simulink model "Copy_of_Pacemaker_images"  (R2022a)
settings: Solver=FixedStepAuto  StartTime=0.0  StopTime=40  FixedStep=1e-3  RelTol=1e-3  EnableMultiTasking=on
undefined symbols (not defined in the file or in its folder): ARP, ATR_Amplitude, ATR_CMP_DETECT, ATR_Pulse_Width, ATR_Sensitivity, D10, D11, D12, D13, D2, D3, D4, D5, D6, D7, D8, D9, Hecate_delayEnd, Hecate_delayOff, Hecate_DELAYOFF, Hecate_delayOn, Hecate_DELAYON, Hecate_HEARTFAIL, Hecate_MODE, LRL, Mode, PTA0, PTA1, PTA2, PTB23, PTB9, PTC2, PTC3, PTC4, PTD0, PTD1, PTD2, PTD3, VENT_Amplitude, VENT_CMP_DETECT, VENT_Pulse_Width, VENT_Sensitivity, VRP
libraries: frdmk64flib x15
settings Model: ExtModeTrigDuration=5  Creator=akshayjacob  LastModifiedBy=fedformi_new
settings DataIOCC: SaveFormat=Array  ReturnWorkspaceOutputs=off
settings OptimizationCC: DefaultParameterBehavior=Inlined  EnhancedBackFolding=on  PassReuseOutputArgsAs=Individual arguments  ZeroExternalMemoryAtStartup=off  ZeroInternalMemoryAtStartup=off  MaxStackSize=64  OptimizeBlockOrder=speed  DifferentSizesBufferReuse=on  OptimizationCustomize=off  EfficientTunableParamExpr=on
settings DebuggingCC: ParameterTunabilityLossMsg=error  UnconnectedInputMsg=warning  UnconnectedOutputMsg=warning  UnconnectedLineMsg=warning
settings HardwareCC: ProdBitPerPointer=32  ProdBitPerSizeT=32  ProdBitPerPtrDiffT=32  ProdLargestAtomicInteger=Long  ProdLargestAtomicFloat=Double  ProdWordSize=32  ProdHWDeviceType=ARM Compatible->ARM Cortex
settings SFSimCC: MATLABDynamicMemAlloc=off
settings RTWCC: SystemTargetFile=ert.tlc  TemplateMakefile=ert_default_tmf  Toolchain=GNU Tools for ARM Embedded Processors  DLArmComputeVersion=19.05
settings CodeAppCC: ForceParamTrailComments=on  IgnoreCustomStorageClasses=off  OperatorAnnotations=on  SimulinkDataObjDesc=on  SFDataObjDesc=on  InsertBlockDesc=on
settings ERTTargetCC: ERTCustomFileTemplate=example_file_process.tlc

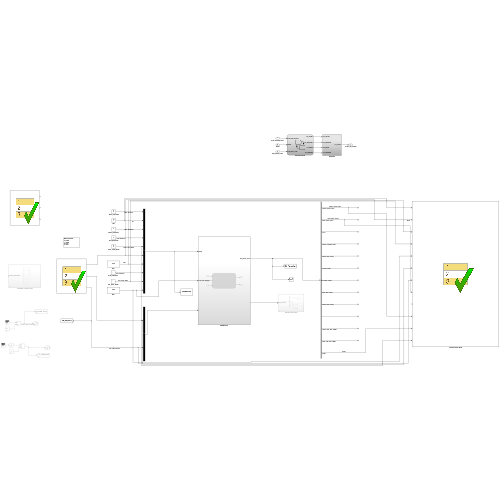
[thumbnail: Simulink's stored preview of the top-level diagram]
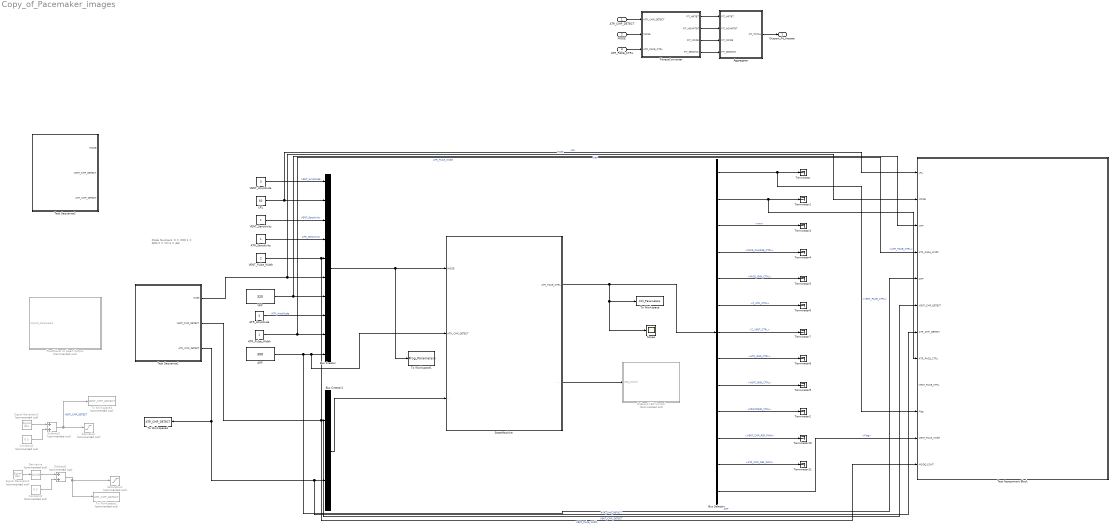
== system Copy_of_Pacemaker_images ==
  note: Mode Numbers:
      |
      | 0 = VOO
      | 1 = AOO
      | 2 = VVI
      | 3 = AAI
  ATR_CMP_DETECT : Inport
  MODE : Inport  Port=2
  ATR_PACE_CTRL : Inport  Port=3
  ARP : Constant  Value=300
  ATR_Amplitude : Constant  Value=3
  ATR_Pulse_Width : Constant
  ATR_Sensitivity : Constant
  Aggregator : Subsystem
  Bus Creator : BusCreator  Inputs=VENT_Amplitude,LRL,VENT_Sensitivity,ATR_Sensitivity,VENT_Pulse_Width,Mode,VRP,ATR_Amplitude,ATR_Pulse_Width,ARP
  Bus Creator1 : BusCreator  Inputs=VENT_CMP_DETECT,ATR_CMP_DETECT
  Bus Selector : BusSelector  OutputSignals=VENT_PACE_CTRL,ATR_PACE_CTRL,nnn,PACE_CHARGE_CTRL,PACE_GND_CTRL,Z_ATR_CTRL,Z_VENT_CTRL,ATR_GND_CTRL,VENT_GND_CTRL,FRONTEND_CTRL,VENT_CMP_REF_PWM,ATR_CMP_REF_PWM,Flag
  Constant1 : Constant  Commented=on  Value=0.5
  Constant2 : Constant  Commented=on  Value=0.5
  Derivative : Derivative  Commented=on
  FitnessConverter : Stateflow chart  TreatAsAtomicUnit=on
  LRL : Constant  Value=60
  OnBoard LED Control : Subsystem  Commented=on
  PaceMaker to Heart Output : Subsystem  Commented=on
  Saturation : Saturate  Commented=on  UpperLimit=1  LowerLimit=0
  Saturation1 : Saturate  Commented=on  UpperLimit=1  LowerLimit=0
  Scope : Scope
  Signal Generator1 : SignalGenerator  Commented=on  Amplitude=1.5  Frequency=1/5
  Signal Generator2 : SignalGenerator  Commented=on  Amplitude=1.5  Frequency=1/5
  StateMachine : Subsystem
  Subtract1 : Sum  Commented=on
  Subtract2 : Sum  Commented=on
  Terminator{,1..11} (12 alike) : Terminator
  Test Assessment Block : Test Sequence  Tag=__SLT_ASMT__  TreatAsAtomicUnit=on
  Test Sequence1 : Test Sequence  TreatAsAtomicUnit=on
  Test Sequence2 : Test Sequence  TreatAsAtomicUnit=on
  To Workspace : ToWorkspace  VariableName=Ctrl_Parameters  SaveFormat=Timeseries  SampleTime=-1
  To Workspace1 : ToWorkspace  VariableName=Prog_Parameters  SaveFormat=Timeseries  SampleTime=-1
  To Workspace2 : ToWorkspace  Commented=on  VariableName=ATR_CMP_DETECT  SaveFormat=Timeseries  SampleTime=-1
  To Workspace3 : ToWorkspace  Commented=on  VariableName=VENT_CMP_DETECT  SaveFormat=Timeseries  SampleTime=-1
  To Workspace4 : ToWorkspace  VariableName=ATR_CMP_DETECT  SaveFormat=Timeseries  SampleTime=-1
  VENT_Amplitude : Constant  Value=3
  VENT_Pulse_Width : Constant  Value=2
  VENT_Sensitivity : Constant
  VRP : Constant  Value=320
  Outport_Fit_Hecate : Outport
  wires:
  Bus Creator/1 -> To Workspace1/1, StateMachine/1(MODE)
  StateMachine/2(.  .  .) -> OnBoard LED Control/1(LED_Control)
  Bus Creator1/1 -> StateMachine/3(. . .)
  VRP/1 -> Test Assessment Block/3(VRP), Bus Creator/7  "VRP"
  ATR_Sensitivity/1 -> Bus Creator/4  "ATR_Sensitivity"
  ATR_Pulse_Width/1 -> Test Assessment Block/4(ATR_Pulse_Width), Bus Creator/9  "ATR_Pulse_Width"
  LRL/1 -> Test Assessment Block/1(LRL), Bus Creator/2  "LRL"
  ATR_Amplitude/1 -> Bus Creator/8  "ATR_Amplitude"
  ARP/1 -> Test Assessment Block/5(ARP), StateMachine/2(ATR_CMP_DETECT), Bus Creator/10  "ARP"
  VENT_Sensitivity/1 -> Bus Creator/3  "VENT_Sensitivity"
  VENT_Amplitude/1 -> Bus Creator/1  "VENT_Amplitude"
  VENT_Pulse_Width/1 -> Test Assessment Block/12(MODE_CONT), Bus Creator/5  "VENT_Pulse_Width"
  Test Sequence1/1(Mode) -> Test Assessment Block/2(MODE), Bus Creator/6  "Mode"
  Subtract1/1 -> Saturation1/1, To Workspace2/1
  Signal Generator2/1 -> Subtract2/1
  Test Sequence1/2(VENT_CMP_DETECT) -> Test Assessment Block/6(VENT_CMP_DETECT), Bus Creator1/1  "VENT_CMP_DETECT"
  Constant1/1 -> Subtract1/2
  Constant2/1 -> Subtract2/2
  Test Sequence1/3(ATR_CMP_DETECT) -> To Workspace4/1, Bus Creator1/2, Test Assessment Block/7(ATR_CMP_DETECT)  "ATR_CMP_DETECT"
  Subtract2/1 -> Saturation/1, To Workspace3/1  "VENT_CMP_DETECT"
  Derivative/1 -> Subtract1/1
  Signal Generator1/1 -> Derivative/1
  Bus Selector/12 -> Terminator11/1  "<ATR_CMP_REF_PWM>"
  Bus Selector/3 -> Terminator3/1  "<nnn>"
  Bus Selector/7 -> Terminator7/1  "<Z_VENT_CTRL>"
  Bus Selector/10 -> Terminator2/1  "<FRONTEND_CTRL>"
  Bus Selector/8 -> Terminator8/1  "<ATR_GND_CTRL>"
  StateMachine/1(ATR_PACE_CTRL) -> Bus Selector/1, Scope/1, To Workspace/1
  Bus Selector/1 -> Test Assessment Block/10(Flag), Terminator/1  "<VENT_PACE_CTRL>"
  Bus Selector/5 -> Terminator5/1  "<PACE_GND_CTRL>"
  Bus Selector/9 -> Terminator9/1  "<VENT_GND_CTRL>"
  Bus Selector/2 -> Test Assessment Block/8(ATR_PACE_CTRL), Terminator1/1  "<ATR_PACE_CTRL>"
  Bus Selector/11 -> Terminator10/1  "<VENT_CMP_REF_PWM>"
  Bus Selector/6 -> Terminator6/1  "<Z_ATR_CTRL>"
  Bus Selector/4 -> Terminator4/1  "<PACE_CHARGE_CTRL>"
  Bus Selector/13 -> Test Assessment Block/11(VENT_Pulse_Width)  "<Flag>"
  FitnessConverter/2(FIT_NOHRTBT) -> Aggregator/2(FIT_NOHRTBT)
  FitnessConverter/3(FIT_MODE) -> Aggregator/3(FIT_MODE)
  Aggregator/1(FIT_TOTAL) -> Outport_Fit_Hecate/1
  FitnessConverter/1(FIT_HRTBT) -> Aggregator/1(FIT_HRTBT)
  FitnessConverter/4(FIT_SENSING) -> Aggregator/4(FIT_SENSING)
  ATR_CMP_DETECT/1 -> FitnessConverter/1(ATR_CMP_DETECT)
  MODE/1 -> FitnessConverter/2(MODE)
  ATR_PACE_CTRL/1 -> FitnessConverter/3(ATR_PACE_CTRL)

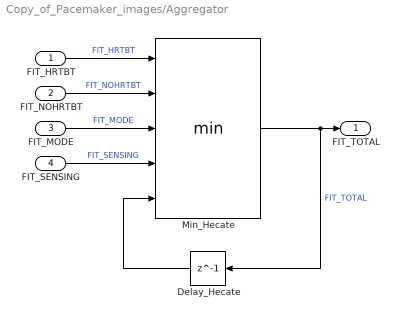
== system Copy_of_Pacemaker_images/Aggregator ==
  FIT_HRTBT : Inport
  FIT_NOHRTBT : Inport  Port=2
  FIT_MODE : Inport  Port=3
  FIT_SENSING : Inport  Port=4
  Delay_Hecate : Delay  DelayLength=1  InitialCondition=Inf
  Min_Hecate : MinMax  Inputs=5
  FIT_TOTAL : Outport
  wires:
  FIT_NOHRTBT/1 -> Min_Hecate/2  "FIT_NOHRTBT"
  FIT_MODE/1 -> Min_Hecate/3  "FIT_MODE"
  Delay_Hecate/1 -> Min_Hecate/5
  FIT_HRTBT/1 -> Min_Hecate/1  "FIT_HRTBT"
  Min_Hecate/1 -> FIT_TOTAL/1, Delay_Hecate/1  "FIT_TOTAL"
  FIT_SENSING/1 -> Min_Hecate/4  "FIT_SENSING"

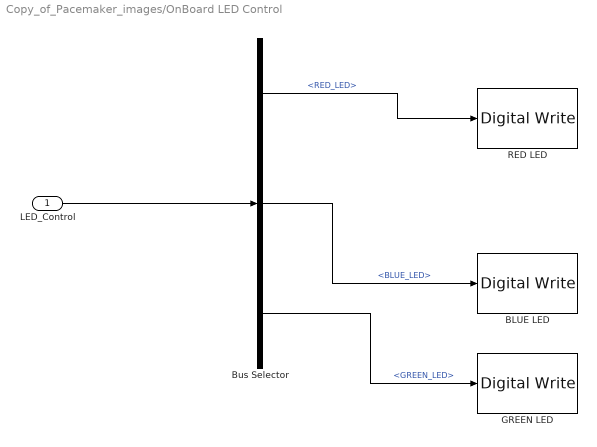
== system Copy_of_Pacemaker_images/OnBoard LED Control ==
  LED_Control : Inport
  BLUE LED : frdmk64flib/Digital Write  Whichpin=BLUE_LED
  Bus Selector : BusSelector  OutputSignals=RED_LED,BLUE_LED,GREEN_LED
  GREEN LED : frdmk64flib/Digital Write  Whichpin=GREEN_LED
  RED LED : frdmk64flib/Digital Write  Whichpin=RED_LED
  wires:
  LED_Control/1 -> Bus Selector/1
  Bus Selector/1 -> RED LED/1  "<RED_LED>"
  Bus Selector/2 -> BLUE LED/1  "<BLUE_LED>"
  Bus Selector/3 -> GREEN LED/1  "<GREEN_LED>"

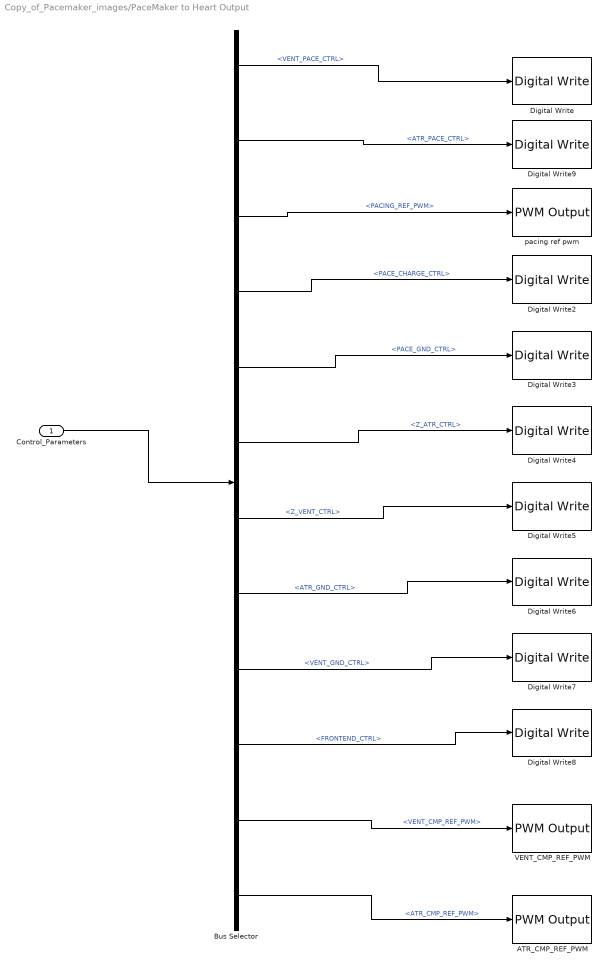
== system Copy_of_Pacemaker_images/PaceMaker to Heart Output ==
  Control_Parameters : Inport
  ATR_CMP_REF_PWM : frdmk64flib/PWM Output  Whichpin=PTC2 (D6)  InitialFrequency=2000  InitialDutyCycle=0
  Bus Selector : BusSelector  OutputSignals=VENT_PACE_CTRL,ATR_PACE_CTRL,PACING_REF_PWM,PACE_CHARGE_CTRL,PACE_GND_CTRL,Z_ATR_CTRL,Z_VENT_CTRL,ATR_GND_CTRL,VENT_GND_CTRL,FRONTEND_CTRL,VENT_CMP_REF_PWM,ATR_CMP_REF_PWM
  Digital Write : frdmk64flib/Digital Write  Whichpin=PTC4 (D9)
  Digital Write2 : frdmk64flib/Digital Write  Whichpin=PTB9 (D2)
  Digital Write3 : frdmk64flib/Digital Write  Whichpin=PTD0 (D10)
  Digital Write4 : frdmk64flib/Digital Write  Whichpin=PTB23 (D4)
  Digital Write5 : frdmk64flib/Digital Write  Whichpin=PTC3 (D7)
  Digital Write6 : frdmk64flib/Digital Write  Whichpin=PTD2 (D11)
  Digital Write7 : frdmk64flib/Digital Write  Whichpin=PTD3 (D12)
  Digital Write8 : frdmk64flib/Digital Write  Whichpin=PTD1 (D13)
  Digital Write9 : frdmk64flib/Digital Write  Whichpin=PTA0 (D8)
  VENT_CMP_REF_PWM : frdmk64flib/PWM Output  Whichpin=PTA1 (D3)  InitialFrequency=2000  InitialDutyCycle=0
  pacing ref pwm : frdmk64flib/PWM Output  Whichpin=PTA2 (D5)  InitialFrequency=2000  InitialDutyCycle=0
  wires:
  Control_Parameters/1 -> Bus Selector/1
  Bus Selector/1 -> Digital Write/1  "<VENT_PACE_CTRL>"
  Bus Selector/3 -> pacing ref pwm/1  "<PACING_REF_PWM>"
  Bus Selector/4 -> Digital Write2/1  "<PACE_CHARGE_CTRL>"
  Bus Selector/5 -> Digital Write3/1  "<PACE_GND_CTRL>"
  Bus Selector/6 -> Digital Write4/1  "<Z_ATR_CTRL>"
  Bus Selector/7 -> Digital Write5/1  "<Z_VENT_CTRL>"
  Bus Selector/8 -> Digital Write6/1  "<ATR_GND_CTRL>"
  Bus Selector/9 -> Digital Write7/1  "<VENT_GND_CTRL>"
  Bus Selector/10 -> Digital Write8/1  "<FRONTEND_CTRL>"
  Bus Selector/2 -> Digital Write9/1  "<ATR_PACE_CTRL>"
  Bus Selector/11 -> VENT_CMP_REF_PWM/1  "<VENT_CMP_REF_PWM>"
  Bus Selector/12 -> ATR_CMP_REF_PWM/1  "<ATR_CMP_REF_PWM>"

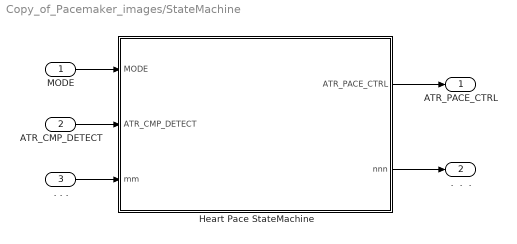
== system Copy_of_Pacemaker_images/StateMachine ==
  MODE : Inport
  ATR_CMP_DETECT : Inport  Port=2
  . . . : Inport  Port=3
  Heart Pace StateMachine : Stateflow chart  TreatAsAtomicUnit=on
  ATR_PACE_CTRL : Outport
  .  .  . : Outport  Port=2
  wires:
  MODE/1 -> Heart Pace StateMachine/1(MODE)
  ATR_CMP_DETECT/1 -> Heart Pace StateMachine/2(ATR_CMP_DETECT)
  . . ./1 -> Heart Pace StateMachine/3(mm)
  Heart Pace StateMachine/1(ATR_PACE_CTRL) -> ATR_PACE_CTRL/1
  Heart Pace StateMachine/2(nnn) -> .  .  ./1

== stateflow chart Copy_of_Pacemaker_images/FitnessConverter ==
  state MODE_SELECTION
    FIT_HRTBT = Inf;
    FIT_NOHRTBT = Inf;
    FIT_MODE = Inf;
    FIT_SENSING = Inf;
    state MODE_3
      FIT_HRTBT = Inf;
      FIT_NOHRTBT = Inf;
      FIT_MODE = Inf;
      FIT_SENSING = Inf;
      state NO_HEARTBEAT
        FIT_HRTBT = Inf;
        FIT_NOHRTBT = 0-(et);
        FIT_MODE = Inf;
        FIT_SENSING = Inf;
      state HEARTBEAT
        FIT_HRTBT = 1;
        FIT_NOHRTBT = Inf;
        FIT_MODE = Inf;
        FIT_SENSING = Inf;
      state SENSING
        FIT_HRTBT = Inf;
        FIT_NOHRTBT = Inf;
        FIT_MODE = Inf;
        FIT_SENSING = 60/LRL-et;
      (default) -> SENSING
      NO_HEARTBEAT -> SENSING : [ATR_CMP_DETECT == true || ...
          |  ATR_PACE_CTRL == true]
      SENSING -> NO_HEARTBEAT [order 2] : [et > 60/LRL]
      SENSING -> HEARTBEAT [order 1] : [ATR_CMP_DETECT == true || ...
          |  ATR_PACE_CTRL == true]
      HEARTBEAT -> SENSING : [true]
    state ELSE
      FIT_HRTBT = Inf;
      FIT_NOHRTBT = Inf;
      FIT_MODE = 3.5-(MODE_CONT);
      FIT_SENSING = Inf;
    (default) -> (junction 4)
    (junction 4) -> ELSE [order 2]
    (junction 4) -> MODE_3 [order 1] : [(MODE == 3)]
    ELSE -> (junction 4) : [((MODE == 3))]
    MODE_3 -> (junction 4) : [~((MODE == 3))]
  (default) -> MODE_SELECTION
  data: ATR_CMP_DETECT input; MODE input; ATR_PACE_CTRL input; FIT_HRTBT output; FIT_NOHRTBT output; FIT_MODE output; MODE_CONT local; LRL local; FIT_SENSING output

== stateflow chart Copy_of_Pacemaker_images/Test Assessment Block ==
  state Complete
    state Run
      state AAI
        state AAI_Refractory
          verify(ATR_PACE_CTRL==0)
          settings: description=|
              | after(ARP-(ATR_Pulse_Width ...
              | *Flag),msec)
        state AAI_Sensing
          verify(ATR_PACE_CTRL==0)
          settings: description=after(60000/LRL-ARP, msec)
        state AAI_Pacing
          verify(ATR_PACE_CTRL==1);
          settings: description=after(ATR_Pulse_Width,msec)
        AAI_Pacing -> (junction 603) : [
            | et > (ATR_Pulse_Width)/1000
            | ]
        (default) -> AAI_Refractory
        (junction 601) -> AAI_Refractory
        AAI_Refractory -> AAI_Sensing : [
            | et > (ARP-(ATR_Pulse_Width ...
            | *Flag))/1000
            | ]
        AAI_Sensing -> AAI_Refractory [order 1] : [
            | [(ATR_CMP_DETECT == 1)]
            | ]
        AAI_Sensing -> AAI_Pacing [order 2] : [
            | et > (60000/LRL-ARP)/1000
            | ]
        (junction 603) -> (junction 601)
      state VVI
        state VVI_REFRACTORY
          verify(VENT_PACE_CTRL==0);
          settings: description=after(VRP - (VENT_Pulse_Width * Flag-1),msec)
        state VVI_SENSE
          verify(VENT_PACE_CTRL==0);
          settings: description=after(60000/LRL - VRP, msec)
        state VVI_PACING
          verify(VENT_PACE_CTRL==1);
          settings: description=after(VENT_Pulse_Width,msec)
        VVI_PACING -> (junction 611) : [
            | et > (VENT_Pulse_Width)/1000
            | ]
        (default) -> VVI_REFRACTORY
        (junction 609) -> VVI_REFRACTORY
        VVI_REFRACTORY -> VVI_SENSE : [
            | et > (VRP - (VENT_Pulse_Width * Flag-1))/1000
            | ]
        VVI_SENSE -> VVI_REFRACTORY [order 2] : [
            | VENT_CMP_DETECT == 1
            | ]
        VVI_SENSE -> VVI_PACING [order 1] : [
            | et > (60000/LRL - VRP)/1000
            | ]
        (junction 611) -> (junction 609)
      state default
      Run -> (junction 557)
      (default) -> (junction 557)
      (junction 557) -> (junction 558) [order 1] : [Mode == 3
          | ]
      (junction 558) -> AAI [order 1] : [~in(Complete.Run.AAI)]
      (junction 557) -> (junction 574) [order 2]
      (junction 558) -> (junction 561) [order 2]
      (junction 574) -> (junction 575) [order 1] : [Mode ==2
          | ]
      (junction 575) -> VVI [order 1] : [~in(Complete.Run.VVI)]
      (junction 575) -> (junction 578) [order 2]
      (junction 590) -> (junction 591)
      (junction 591) -> default [order 1] : [~in(Complete.Run.default)]
      (junction 591) -> (junction 594) [order 2]
      (junction 574) -> (junction 590) [order 2]
    (default) -> Run
  state Partial
    state Mode_selection
      state Mode_3
        state Sensing
          verify(et <= 60/LRL)
        state Heartbeat
          verify(true)
        state No_heartbeat
          verify(false)
        (junction 677) -> (junction 660)
        (default) -> Sensing
        (junction 660) -> Sensing
        Sensing -> (junction 672) [order 2] : [
            | et >= 60/LRL
            | ]
        (junction 672) -> (junction 652)
        Sensing -> Heartbeat [order 1] : [
            | ATR_CMP_DETECT == true || ...
            |  ATR_PACE_CTRL == true
            | ]
        Heartbeat -> Sensing : [
            | true
            | ]
        (junction 652) -> No_heartbeat
        No_heartbeat -> (junction 677) : [
            | ATR_CMP_DETECT == true || ...
            |  ATR_PACE_CTRL == true
            | ]
      state Else
        verify(MODE_CONT <= 3.5)
      (default) -> (junction 627)
      Mode_selection -> (junction 627)
      (junction 627) -> (junction 628) [order 1] : [(MODE == 3)
          | ]
      (junction 628) -> Mode_3 [order 1] : [~in(Partial.Mode_selection.Mode_3)]
      (junction 627) -> (junction 636) [order 2]
      (junction 628) -> (junction 631) [order 2]
      (junction 636) -> (junction 637)
      (junction 637) -> Else [order 1] : [~in(Partial.Mode_selection.Else)]
      (junction 637) -> (junction 640) [order 2]
    (default) -> Mode_selection
  (default) -> Complete [order 1] : [Active_Scenario_Index == 1]
  (default) -> Partial [order 2] : {assert(Active_Scenario_Index == 2,'The value of Scenario Parameter ''Active_Scenario_Index'' is not valid. Use the index of the scenario to specify it.')}
  data: LRL input double size=[1]; MODE input double size=[1]; VRP input size=[1]; ATR_Pulse_Width input double size=[1]; ARP input size=[1]; VENT_CMP_DETECT input size=[1, 1]; ATR_CMP_DETECT input size=[1, 1]; ATR_PACE_CTRL input double size=[1]; VENT_PACE_CTRL input double size=[1]; Flag input; VENT_Pulse_Width input; Active_Scenario_Index parameter =2; MODE_CONT input

== stateflow chart Copy_of_Pacemaker_images/Test Sequence1 ==
  settings: updateMethod=DISCRETE  sampleTime=0.001
  state Initialize
    %. . .
    ATR_CMP_DETECT=false;
  state AAI_Mode_3
    Mode=3;
    state AAI_Mode_3_OFF
      ATR_CMP_DETECT=false;
    state AAI_Mode_3_ON
      ATR_CMP_DETECT=true;
    (default) -> AAI_Mode_3_OFF
    AAI_Mode_3_OFF -> AAI_Mode_3_ON : [
        | after(3+...
        | Hecate_delayOn,sec)
        | ]
    AAI_Mode_3_ON -> AAI_Mode_3_OFF : [
        | after(1+...
        | Hecate_delayOff,sec)
        | ]
  state END
    ATR_CMP_DETECT=false;
  (default) -> Initialize
  Initialize -> AAI_Mode_3 : [
      | true
      | ]
  AAI_Mode_3 -> END : [
      | after(20+...
      | Hecate_delayEnd,sec)
      | ]
  data: Mode output double size=[1]; VENT_CMP_DETECT output boolean size=[1, 1]; ATR_CMP_DETECT output boolean size=[1, 1]; Hecate_delayEnd parameter; Hecate_delayOn parameter; Hecate_delayOff parameter

== stateflow chart Copy_of_Pacemaker_images/Test Sequence2 ==
  settings: updateMethod=DISCRETE  sampleTime=0.001
  state Parametrized
    state AAI_Mode_3
      MODE = Hecate_MODE;
      . . .
      state AAI_Mode_3_OFF
        ATR_CMP_DETECT = false;
      state AAI_Mode_3_ON
        ATR_CMP_DETECT = true;
      (default) -> Parametrized.AAI_Mode_3.AAI_Mode_3_OFF
      Parametrized.AAI_Mode_3.AAI_Mode_3_OFF -> Parametrized.AAI_Mode_3.AAI_Mode_3_ON : [
          | after(2+...
          | Hecate_DELAYON,sec)
          | ]
      Parametrized.AAI_Mode_3.AAI_Mode_3_ON -> Parametrized.AAI_Mode_3.AAI_Mode_3_OFF : [
          | after(0.05+...
          | Hecate_DELAYOFF,sec)
          | ]
    state END
      ATR_CMP_DETECT = false;
    (default) -> Parametrized.AAI_Mode_3
    Parametrized.AAI_Mode_3 -> Parametrized.END : [
        | after(...
        | Hecate_HEARTFAIL,sec)
        | ]
  state Unparametrized
    state AAI_Mode_3
      MODE = 3;
      . . .
      state AAI_Mode_3_OFF
        ATR_CMP_DETECT = false;
      state AAI_Mode_3_ON
        ATR_CMP_DETECT = true;
      (default) -> Unparametrized.AAI_Mode_3.AAI_Mode_3_OFF
      Unparametrized.AAI_Mode_3.AAI_Mode_3_OFF -> Unparametrized.AAI_Mode_3.AAI_Mode_3_ON : [
          | after(2, sec)
          | ]
      Unparametrized.AAI_Mode_3.AAI_Mode_3_ON -> Unparametrized.AAI_Mode_3.AAI_Mode_3_OFF : [
          | after(0.05, sec)
          | ]
    state END
      ATR_CMP_DETECT = false;
    (default) -> Unparametrized.AAI_Mode_3
    Unparametrized.AAI_Mode_3 -> Unparametrized.END : [
        | after(40, sec)
        | ]
  (default) -> Parametrized [order 1] : [Active_Scenario_Index == 1]
  (default) -> Unparametrized [order 2] : {assert(Active_Scenario_Index == 2,'The value of Scenario Parameter ''Active_Scenario_Index'' is not valid. Use the index of the scenario to specify it.')}
  data: MODE output double size=[1]; VENT_CMP_DETECT output boolean size=[1, 1]; ATR_CMP_DETECT output boolean size=[1, 1]; Hecate_HEARTFAIL parameter; Hecate_DELAYON parameter; Hecate_DELAYOFF parameter; Hecate_MODE parameter; Active_Scenario_Index parameter =1

== stateflow chart Copy_of_Pacemaker_images/StateMachine/Heart Pace StateMachine ==
  state VOO_ChargingState
    entry:
    ATR_PACE_CTRL = 0;
    VENT_PACE_CTRL = 0;
    nnn = VENT_Amplitude/5*100
    PACE_CHARGE_CTRL = 1;
    PACE_GND_CTRL = 1;
    Z_ATR_CTRL = 0;
    Z_VENT_CTRL = 0;
    ATR_GND_CTRL = 0;
    VENT_GND_CTRL = 1;
    BLUE_LED = 0;
    RED_LED = 1;
  state VOO_Pacing
    entry:
    PACE_CHARGE_CTRL = 0;
    PACE_GND_CTRL = 1;
    ATR_GND_CTRL = 0;
    ATR_PACE_CTRL = 0;
    Z_ATR_CTRL = 0;
    Z_VENT_CTRL =0;
    VENT_PACE_CTRL = 1;
    VENT_GND_CTRL = 0;
    nnn = VENT_Amplitude/5*100;
    BLUE_LED=1;
    RED_LED=0;
  state AOO_ChargingState
    entry:
    ATR_PACE_CTRL = 0;
    VENT_PACE_CTRL = 0;
    nnn = mm/5*100
    PACE_CHARGE_CTRL = 1;
    PACE_GND_CTRL = 1;
    Z_ATR_CTRL = 0;
    Z_VENT_CTRL = 0;
    ATR_GND_CTRL = 1;
    VENT_GND_CTRL = 0;
    BLUE_LED = 0;
    RED_LED = 1;
  state AOO_Pacing
    entry:
    PACE_CHARGE_CTRL = 0;
    PACE_GND_CTRL = 1;
    ATR_GND_CTRL = 0;
    ATR_PACE_CTRL = 1;
    Z_ATR_CTRL = 0;
    Z_VENT_CTRL =0;
    VENT_PACE_CTRL = 0;
    VENT_GND_CTRL = 0;
    nnn = mm/5*100;
    BLUE_LED=1;
    RED_LED=0;
  state MAIN
    entry:
    PACE_CHARGE_CTRL = 0;
    VENT_PACE_CTRL = 0;
    ATR_PACE_CTRL = 0;
    PACE_GND_CTRL = 0;
    ATR_GND_CTRL = 0;
    VENT_GND_CTRL = 0;
    Z_ATR_CTRL = 0;
    Z_VENT_CTRL = 0;
    FRONTEND_CTRL = 0;
    RED_LED = 0;
    BLUE_LED=0;
    Flag = 0;
  state VVI_Sensing
    entry:
    BLUE_LED = 0;
    RED_LED = 0;
    GREEN_LED = 1;
    FRONTEND_CTRL = 1;
    Flag = 0;
  state VVI_Refactory
    entry:
    ATR_PACE_CTRL = 0;
    VENT_PACE_CTRL = 0;
    nnn = VENT_Amplitude/5*100;
    PACE_CHARGE_CTRL = 1;
    PACE_GND_CTRL = 1;
    Z_ATR_CTRL = 0;
    Z_VENT_CTRL = 0;
    ATR_GND_CTRL = 0;
    VENT_GND_CTRL = 1;
    FRONTEND_CTRL = 1;
    VENT_CMP_REF_PWM = VENT_Sensitivity/5*100;
    BLUE_LED = 0;
    RED_LED = 1;
    GREEN_LED = 0;
  state VVI_Pacing
    entry:
    FRONTEND_CTRL = 0;
    PACE_CHARGE_CTRL = 0;
    PACE_GND_CTRL = 1;
    ATR_GND_CTRL = 0;
    ATR_PACE_CTRL = 0;
    Z_ATR_CTRL = 0;
    Z_VENT_CTRL =0;
    VENT_PACE_CTRL = 1;
    VENT_GND_CTRL = 0;
    nnn = VENT_Amplitude/5*100;
    BLUE_LED = 1;
    RED_LED = 0;
    GREEN_LED = 0;
    Flag = 1;
  state AAI_Sensing
    entry:
    BLUE_LED = 0;
    RED_LED = 0;
    GREEN_LED = 1;
    Flag = 0;
  note: Subtract PW from this based on previous event
      | -sense heart rate: dont (no pulsewith done by pacemaker)
      | -pulsed rate: subtract PW
      |  vrp-(pulsewith*flag)
  state AAI_Refactory
    entry:
    ATR_PACE_CTRL = 0;
    VENT_PACE_CTRL = 0;
    nnn = mm/5*100;
    PACE_CHARGE_CTRL = 1;
    PACE_GND_CTRL = 1;
    Z_ATR_CTRL = 0;
    Z_VENT_CTRL = 0;
    ATR_GND_CTRL = 1;
    VENT_GND_CTRL = 0;
    FRONTEND_CTRL = 1;
    ATR_CMP_REF_PWM= ATR_Sensitivity/5*100;
    BLUE_LED = 0;
    RED_LED = 1;
    GREEN_LED = 1;
  state AAI_Pacing
    entry:
    FRONTEND_CTRL = 0;
    PACE_CHARGE_CTRL = 0;
    PACE_GND_CTRL = 1;
    ATR_GND_CTRL = 0;
    ATR_PACE_CTRL = 1;
    Z_ATR_CTRL = 0;
    Z_VENT_CTRL =0;
    VENT_PACE_CTRL = 0;
    VENT_GND_CTRL = 0;
    nnn = mm/5*100;
    BLUE_LED = 1;
    RED_LED = 0;
    GREEN_LED = 0;
    Flag = 1;
  VOO_ChargingState -> VOO_Pacing : after((60000/LRL) - VENT_Pulse_Width,msec)
  MAIN -> VOO_ChargingState [order 1] : [MODE == 0]
  VOO_Pacing -> VOO_ChargingState : after(VENT_Pulse_Width, msec)
  (default) -> MAIN
  AOO_ChargingState -> AOO_Pacing : after((60000/LRL) - ATR_Pulse_Width,msec)
  MAIN -> AOO_ChargingState [order 4] : [MODE == 1]
  AOO_Pacing -> AOO_ChargingState : after(ATR_Pulse_Width, msec)
  MAIN -> VVI_Refactory [order 2] : [MODE == 2]
  MAIN -> AAI_Refactory [order 3] : [MODE==3]
  VVI_Refactory -> VVI_Sensing : after(VRP - (VENT_Pulse_Width * Flag),msec)
  VVI_Sensing -> VVI_Pacing [order 2] : after(60000/LRL - VRP, msec)
  VVI_Sensing -> VVI_Refactory [order 1] : [(VENT_CMP_DETECT == 1)]
  VVI_Pacing -> VVI_Refactory : after(VENT_Pulse_Width,msec)
  AAI_Refactory -> AAI_Sensing : after(ARP  - (ATR_Pulse_Width * Flag),msec)
  AAI_Sensing -> AAI_Pacing [order 2] : after(60000/LRL - ARP, msec)
  AAI_Sensing -> AAI_Refactory [order 1] : [ATR_CMP_DETECT >= 1]
  AAI_Pacing -> AAI_Refactory : after(ATR_Pulse_Width,msec)
  data: MODE input; ATR_PACE_CTRL output; nnn output; ATR_CMP_DETECT input; mm input
